simulink model "mode_pan_controller"  (R2017a)
settings: Solver=VariableStepAuto  StartTime=0.0  StopTime=10.0  RelTol=1e-3
libraries: simulink x1
settings Model: Creator=mini  LastModifiedBy=mini

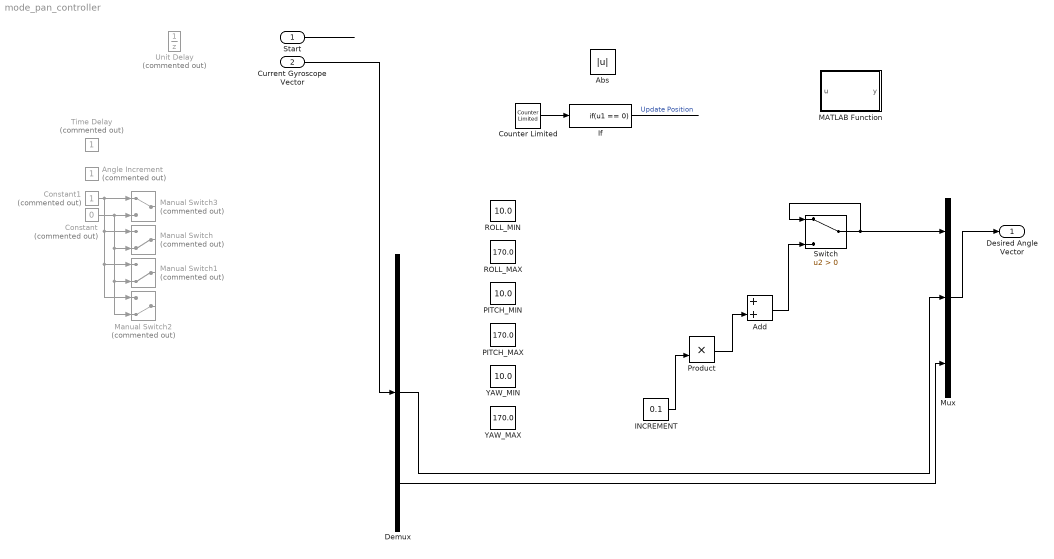
== system mode_pan_controller ==
  Start : Inport
  Current Gyroscope Vector : Inport  Port=2
  Abs : Abs
  Add : Sum
  Angle Increment : Constant  Commented=on
  Constant : Constant  Commented=on  Value=0
  Constant1 : Constant  Commented=on
  Counter Limited : simulink/Sources/Counter Limited  uplimit=7  tsamp=-1
  Demux : Demux  Outputs=3
  INCREMENT : Constant  Value=0.1
  If : If  IfExpression=u1 == 0  ShowElse=off
  MATLAB Function : MATLAB Function  TreatAsAtomicUnit=on
  Manual Switch : ManualSwitch  Commented=on  CurrentSetting=0
  Manual Switch1 : ManualSwitch  Commented=on  CurrentSetting=0
  Manual Switch2 : ManualSwitch  Commented=on  CurrentSetting=0
  Manual Switch3 : ManualSwitch  Commented=on
  Mux : Mux  Inputs=3
  PITCH_MAX : Constant  Value=170.0
  PITCH_MIN : Constant  Value=10.0
  Product : Product
  ROLL_MAX : Constant  Value=170.0
  ROLL_MIN : Constant  Value=10.0
  Switch : Switch  Criteria=u2 > Threshold
  Time Delay : Constant  Commented=on
  Unit Delay : UnitDelay  Commented=on  SampleTime=-1
  YAW_MAX : Constant  Value=170.0
  YAW_MIN : Constant  Value=10.0
  Desired Angle Vector : Outport
  wires:
  Current Gyroscope Vector/1 -> Demux/1
  Constant1/1 -> Manual Switch3/1, Manual Switch/1, Manual Switch2/1, Manual Switch1/1
  Constant/1 -> Manual Switch3/2, Manual Switch2/2, Manual Switch1/2, Manual Switch/2
  Start/1 -> ?
  Counter Limited/1 -> If/1
  If/1 -> ?  "Update Position"
  INCREMENT/1 -> Product/2
  Product/1 -> Add/2
  Switch/1 -> Mux/1, Switch/1
  Add/1 -> Switch/3
  ? -> Switch/2  "UpdatePosition"
  Mux/1 -> Desired Angle Vector/1
  Demux/2 -> Mux/2
  Demux/3 -> Mux/3

== matlab function mode_pan_controller/MATLAB Function ==
  data: u input; y output
function y = fcn(u)
    %{
    Description of how this works
    incrementer = 0.1
    min = 10
    max = 170
    currAngle = ...
    tolerance = ...

    desired = 0
    while( abs(currAngle - desired) > tolerance ) 
        // wait for starting position to be found
    // pan back
    while(1)
        if abs(currAngle - desiredAngle) < tolerance 
            desired = currAngle + incrmenter
        end
    end while
    // pan one way
    while(1)
        if abs(currAngle - desiredAngle) < tolerance 
            desired = currAngle - incrmenter
        end
    end while

    // do other axis
    // stuff
    %}
y = u;
